simulink model "deneme"  (R2014a)
settings: Solver=ode1  SolverMode=SingleTasking  StartTime=0.0  StopTime=10.0  FixedStep=0.001  RelTol=1e-3
settings Model: Creator=robotlab  LastModifiedBy=robotlab
settings RTWCC: SystemTargetFile=zenom.tlc  TemplateMakefile=zenom.tmf  Description=Linux / Zenom Real-Time Target  GenerateReport=on  ProcessScript=zenom_make_rtw_hook  LaunchReport=on
settings GRTTargetCC: CombineOutputUpdateFcns=off  GRTInterface=on  RTWCAPISignals=on  RTWCAPIParams=on

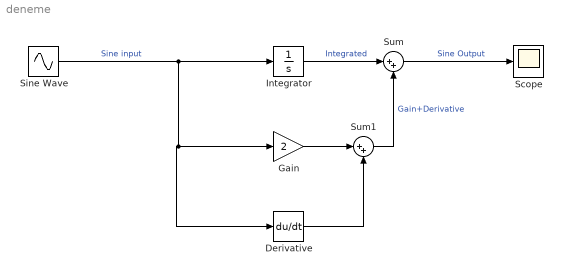
== system deneme ==
  Derivative : Derivative
  Gain : Gain  Gain=2
  Integrator : Integrator
  Scope : Scope
  Sine Wave : Sin  SampleTime=0
  Sum : Sum  Inputs=|++
  Sum1 : Sum  Inputs=|++
  wires:
  Sine Wave/1 -> Derivative/1, Gain/1, Integrator/1  "Sine input"
  Sum/1 -> Scope/1  "Sine Output"
  Sum1/1 -> Sum/2  "Gain+Derivative"
  Gain/1 -> Sum1/1
  Derivative/1 -> Sum1/2
  Integrator/1 -> Sum/1  "Integrated"
